simulink model "DC_motor_verified"  (R2017a)
settings: Solver=VariableStepAuto  StartTime=0.0  StopTime=10.0  RelTol=1e-3
values from neighbouring files (symbols this model uses):
  param = zeros(2,1)    [parameter_estimation_script.m]
settings Model: Creator=USER  LastModifiedBy=dell

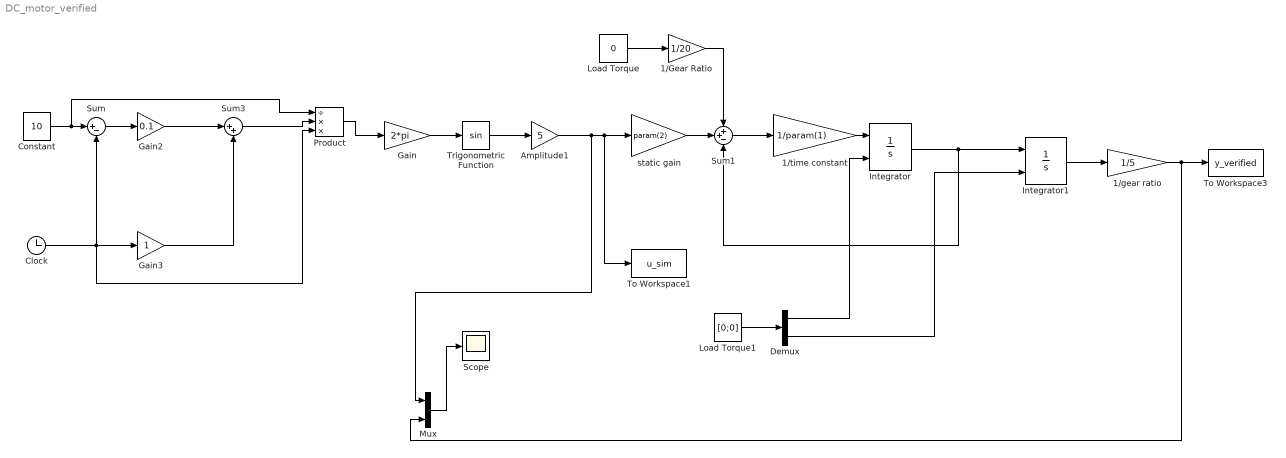
== system DC_motor_verified ==
  1/Gear Ratio : Gain  Gain=1/20
  1/gear ratio : Gain  Gain=1/5
  1/time constant : Gain  Gain=1/param(1)
  Amplitude1 : Gain  Gain=5
  Clock : Clock
  Constant : Constant  Value=10
  Demux : Demux  Outputs=2
  Gain : Gain  Gain=2*pi
  Gain2 : Gain  Gain=0.1
  Gain3 : Gain
  Integrator : Integrator  InitialConditionSource=external
  Integrator1 : Integrator  InitialConditionSource=external
  Load Torque : Constant  Value=0
  Load Torque1 : Constant  Value=[0;0]
  Mux : Mux  Inputs=2
  Product : Product  Inputs=/**
  Scope : Scope
  Sum : Sum  Inputs=|+-
  Sum1 : Sum  Inputs=++-
  Sum3 : Sum  Inputs=|++
  To Workspace1 : ToWorkspace  VariableName=u_sim  SaveFormat=Timeseries  SampleTime=-1
  To Workspace3 : ToWorkspace  VariableName=y_verified  SaveFormat=Timeseries  SampleTime=-1
  Trigonometric Function : Trigonometry
  static gain : Gain  Gain=param(2)
  wires:
  Integrator/1 -> Integrator1/1, Sum1/3
  1/time constant/1 -> Integrator/1
  Sum1/1 -> 1/time constant/1
  Amplitude1/1 -> Mux/1, To Workspace1/1, static gain/1
  Integrator1/1 -> 1/gear ratio/1
  1/gear ratio/1 -> Mux/2, To Workspace3/1
  static gain/1 -> Sum1/2
  1/Gear Ratio/1 -> Sum1/1
  Load Torque/1 -> 1/Gear Ratio/1
  Demux/1 -> Integrator/2
  Demux/2 -> Integrator1/2
  Load Torque1/1 -> Demux/1
  Trigonometric Function/1 -> Amplitude1/1
  Gain/1 -> Trigonometric Function/1
  Product/1 -> Gain/1
  Clock/1 -> Product/3, Gain3/1, Sum/2
  Constant/1 -> Product/1, Sum/1
  Gain2/1 -> Sum3/1
  Sum/1 -> Gain2/1
  Gain3/1 -> Sum3/2
  Sum3/1 -> Product/2
  Mux/1 -> Scope/1
